simulink model "lb682_rtlsdr_rx_am_dsb_sc_costas"  (R2018b)
settings: Solver=VariableStepAuto  StartTime=0.0  StopTime=inf  RelTol=1e-3
PreLoadFcn:
  | % параметры контура ФАПЧ
  | fs=240e3; % частота дискретизации (Гц)
  | A = 1;       % амплитуда входного сигнала
  | T = 1/fs;    % период дискретизации
  | Kp = A/2;   % коэффициент усиления ФД
  | Bn = 1000; % шумовая полоса, Гц
  | Ko = 1;      % коэффициент усиления ГУН (нормирован к fs)
  | d = 0.707;  % демпинг фактор
  | % оценка коэффициентов ПФ
  | K1 = (4*d*Bn*T)/(Ko*Kp*(d+1/(4*d)));
  | K2 = (4*(Bn*T)^2)/(Ko*Kp*(d+1/4*d)^2);
libraries: dsparch4 x2, commsynccomp2 x2, dspsnks4 x1, dspmlti4 x1, sdrrlib x1
settings Model: SimulationMode=accelerator  Creator=Григорий Фокин  LastModifiedBy=Григорий Фокин
settings SFSimCC: SimUseLocalCustomCode=off
settings RTWCC: RTWUseLocalCustomCode=off
settings CodeAppCC: StateflowObjectComments=on

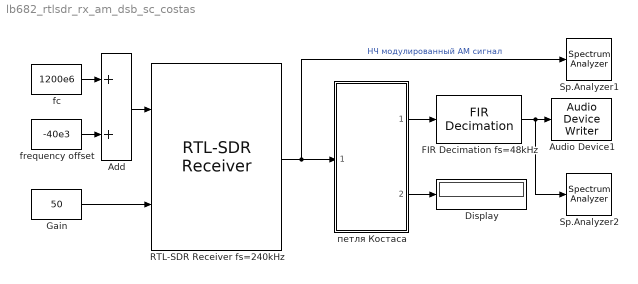
== system lb682_rtlsdr_rx_am_dsb_sc_costas ==
  Add : Sum
  Audio Device1 : dspsnks4/Audio Device Writer  Driver=DirectSound  Device=Default  InheritSampleRate=on  SampleRate=44100  BitDepth=16-bit integer  BufferSize=4096  NumBuffers=10  DefaultOutputChannelMapping=on  OutputChannelMapping=1:2  OutputNumUnderrunSamples=off  DriverIdx=1  DeviceWarnFlag=''
  Display : Display
  FIR Decimation fs=48kHz : dspmlti4/FIR Decimation  FilterSource=Dialog parameters  h=firpm(100, [0 15e3 20e3 (240e3/2)]/(240e3/2), [1 1 0 0], [1 1], 20)  D=5  filtStruct=Direct form  FilterObject=FDECIM  InputProcessing=Columns as channels (frame based)  framing=Allow multirate processing  inputOffset=0  outputBufInitCond=0  roundingMode=Floor  overflowMode=off  firstCoeffDataTypeStr=Inherit: Same word length as input  firstCoeffMin=[]  firstCoeffMax=[]  firstCoeffLastDataTypeStr=Inherit: Same word length as input  outputDataTypeStr=Inherit: Same as accumulator  outputMin=[]  outputMax=[]  outputLastDataTypeStr=Inherit: Same as accumulator
  Gain : Constant  Value=50
  RTL-SDR Receiver fs=240kHz : sdrrlib/RTL-SDR Receiver  IPAddress=0  CenterFrequencySource=Input port  CenterFrequency=102.5e6  GainSource=Input port  Gain=0  ADCRate=240e3  FrequencyCorrection=50  LostSamplesOutputPort=off  LatencyOutputPort=off  OutputDataType=single  FrameLength=4096  EnableBurstMode=off  NumFramesInBurst=20  sobjType=sdrr.internal.SDRRTLReceiverSL  dataUDPPort=-1  ctrlUDPPort=-1  subDeviceList=nosubdev  sdrBlockType=SDRBlockTypeSLT.SDRRxBlock  requester=UNUSED_BY_SFCN  sdrExecutionMode=SDRExecutionModeSLT.ExecModeHW  BypassUserLogic=off  DecimatorSelect=DDC decimator  SourceSelect=RF data  SineAmplitude=16000  EnableInternalClock=off  BypassIQBalance=off  IFBandwidth=40e6  ADCRateSource=Dialog  IntermediateFrequency=0  DecimationFactorSource=Dialog  DecimationFactor=512  RFFrequencyIsTunable=logical(1)  SampleTime=(4096)/(240e3)  IFBandwidthSource=Dialog  SineFrequency=30000  BypassDCBlockingFilter=off  IntermediateFrequencySource=Dialog  IQBalanceCoefficients=64  SkipAllHardwareResetAndInitialization=off  EnableIQCalibrationTable=on  CacheIQCalibrationTable=off  EnableOffsetTuning=off  EnableRTLAGC=off  EnableTestMode=off  EnableTunerAGC=off  FrequencyCorrectionSource=Dialog  NumMLBuffers=128  NumUSBBuffers=16  RTLCrystalFrequency=28800000  TunerCrystalFrequency=28800000
      settings: SourceProductName=Communications System Toolbox Support Package for RTL-SDR Radio  SourceProductBaseCode=RTLSDR
  Sp.Analyzer1 : SpectrumAnalyzer
  Sp.Analyzer2 : SpectrumAnalyzer
  fc : Constant  Value=1200e6
  frequency offset : Constant  Value=-40e3
  петля Костаса : Subsystem  mask{fc=40e3, frame_size=4096}
      mask prompts: fc "Quiescent frequency (Гц)"; frame_size "Размер буфера"
  wires:
  Add/1 -> RTL-SDR Receiver fs=240kHz/1
  fc/1 -> Add/1
  frequency offset/1 -> Add/2
  Gain/1 -> RTL-SDR Receiver fs=240kHz/2
  RTL-SDR Receiver fs=240kHz/1 -> петля Костаса/1(demod_in), Sp.Analyzer1/1  "НЧ модулированный АМ сигнал"
  петля Костаса/1(demod_out) -> FIR Decimation fs=48kHz/1
  FIR Decimation fs=48kHz/1 -> Audio Device1/1, Sp.Analyzer2/1
  петля Костаса/2(freq_out) -> Display/1

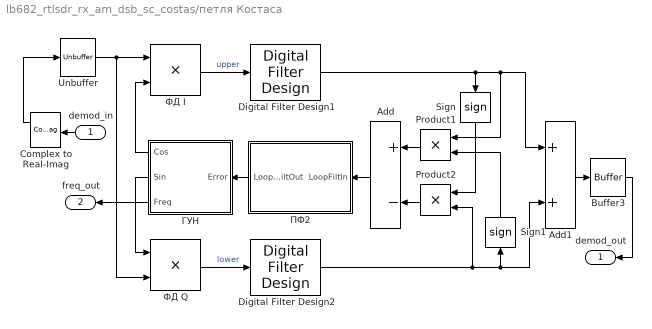
== system lb682_rtlsdr_rx_am_dsb_sc_costas/петля Костаса ==
  demod_in : Inport
  Add : Sum  Inputs=+-
  Add1 : Sum
  Buffer3 : Buffer  N=frame_size  OutputFrames=off
  Complex to Real-Imag : ComplexToRealImag
  Digital Filter Design1 : dsparch4/Digital Filter Design  mwdsp_browser_bugfix_var=off
  Digital Filter Design2 : dsparch4/Digital Filter Design  mwdsp_browser_bugfix_var=off
  Product1 : Product
  Product2 : Product
  Sign : Signum
  Sign1 : Signum
  Unbuffer : Unbuffer
  ГУН : Subsystem  mask(Quadratude VCO){fq=fc, sensitivity=Ko*fs}
      mask prompts: fq "Quiescent Frequency (Hz)"; sensitivity "Sensitivity (Hz/V)"
      mask help: This VCO provides both cosine and sine outputs. The quiescent frequency and sensitivity of the VCO can be defined via the mask (and these apply to both sine and cosine outputs). The block also provides the instantaneous frequency as an output.
  ПФ2 : Subsystem  mask(Loop Filter (Type 2)){K1=K1, K2=K2}
      mask prompts: K1 "K1 (proportional path)"; K2 "K2 (integral path)"
      mask help: This loop filter contains two paths: a proportional path with scaling coefficient K1, and an integral path with scaling coefficient K2.
  ФД I : Product
  ФД Q : Product
  demod_out : Outport
  freq_out : Outport  Port=2
  wires:
  ПФ2/1(LoopFiltOut) -> ГУН/1(Error)
  ГУН/1(Cos) -> ФД I/2
  Unbuffer/1 -> ФД Q/2, ФД I/1
  ГУН/2(Sin) -> ФД Q/1
  demod_in/1 -> Complex to Real-Imag/1
  Complex to Real-Imag/1 -> Unbuffer/1
  Add/1 -> ПФ2/1(LoopFiltIn)
  Product1/1 -> Add/1
  Product2/1 -> Add/2
  ФД I/1 -> Digital Filter Design1/1  "upper"
  ФД Q/1 -> Digital Filter Design2/1  "lower"
  Digital Filter Design1/1 -> Sign/1, Add1/1, Product1/1
  Sign/1 -> Product2/1
  Digital Filter Design2/1 -> Product2/2, Add1/2, Sign1/1
  Sign1/1 -> Product1/2
  Add1/1 -> Buffer3/1
  Buffer3/1 -> demod_out/1
  ГУН/3(Freq) -> freq_out/1

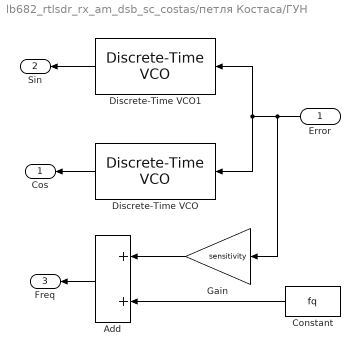
== system lb682_rtlsdr_rx_am_dsb_sc_costas/петля Костаса/ГУН ==
  Error : Inport
  Add : Sum
  Constant : Constant  Value=fq  SampleTime=1/fs
  Discrete-Time VCO : commsynccomp2/Discrete-Time VCO  Ac=1  Fc=fq  Kc=sensitivity  Ph=pi/2  ts=1/fs
      settings: SourceProductName=Communications System Toolbox  SourceProductBaseCode=CM
  Discrete-Time VCO1 : commsynccomp2/Discrete-Time VCO  Ac=1  Fc=fq  Kc=sensitivity  Ph=0  ts=1/fs
      settings: SourceProductName=Communications System Toolbox  SourceProductBaseCode=CM
  Gain : Gain  Gain=sensitivity
  Cos : Outport
  Sin : Outport  Port=2
  Freq : Outport  Port=3
  wires:
  Gain/1 -> Add/1
  Constant/1 -> Add/2
  Add/1 -> Freq/1
  Error/1 -> Discrete-Time VCO/1, Discrete-Time VCO1/1, Gain/1
  Discrete-Time VCO1/1 -> Sin/1
  Discrete-Time VCO/1 -> Cos/1

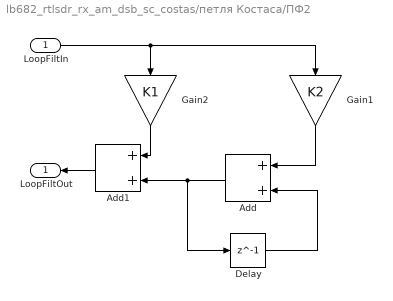
== system lb682_rtlsdr_rx_am_dsb_sc_costas/петля Костаса/ПФ2 ==
  LoopFiltIn : Inport
  Add : Sum
  Add1 : Sum
  Delay : Delay  DelayLength=1
  Gain1 : Gain  Gain=K2
  Gain2 : Gain  Gain=K1
  LoopFiltOut : Outport
  wires:
  Add1/1 -> LoopFiltOut/1
  Delay/1 -> Add/2
  Add/1 -> Delay/1, Add1/2
  LoopFiltIn/1 -> Gain1/1, Gain2/1
  Gain2/1 -> Add1/1
  Gain1/1 -> Add/1
